simulink model "cov_test_model"  (Simulink 7.8)
settings: Solver=VariableStepDiscrete  StartTime=0.0  StopTime=10^-4  RelTol=1e-3
settings Model: Creator=chuh  LastModifiedBy=chuh

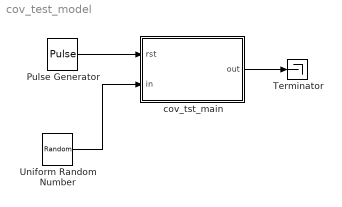
== system cov_test_model ==
  Pulse Generator : DiscretePulseGenerator  PulseType=Time based  Period=10^-5  PulseWidth=5
  Terminator : Terminator
  Uniform Random Number : UniformRandomNumber  Minimum=-128  Maximum=127  SampleTime=10^-6
  cov_tst_main : Subsystem  mask(cov_tst_main){params_samples=1e-6, params_freq=1}
      mask prompts: params_samples "Sample time:"; params_freq "FPGA frequency (MHz):"
      mask help:
      | input rst
      | input in[7:0]
      | output out[7:0]
      mask Help:
      | input rst
      | input in[7:0]
      | output out[7:0]
  wires:
  Pulse Generator/1 -> cov_tst_main/1(rst)
  Uniform Random Number/1 -> cov_tst_main/2(in)
  cov_tst_main/1(out) -> Terminator/1

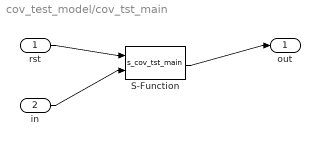
== system cov_test_model/cov_tst_main ==
  rst : Inport  OutDataTypeStr=double  SampleTime=1e-10
  in : Inport  Port=2  OutDataTypeStr=double  SampleTime=1e-10
  S-Function : S-Function  FunctionName=s_cov_tst_main  Parameters=params_samples, params_freq  EnableBusSupport=off
  out : Outport  OutDataTypeStr=uint32  SampleTime=1e-10
  wires:
  rst/1 -> S-Function/1
  in/1 -> S-Function/2
  S-Function/1 -> out/1
